simulink model "Tflex_PIDv1_ISSGP18a"  (R2018a)
settings: Solver=FixedStepDiscrete  StartTime=0.0  StopTime=inf  FixedStep=0.001  RelTol=1e-3  EnableMultiTasking=on
PreLoadFcn:
  | Ts = 0.001;
InitFcn:
  | Ts = 0.001;
values from neighbouring files (symbols this model uses):
  a0 = W_n^3    (= 31006276.6803)    [init_Tflex_PID_ISSGP.m]
  a1 = 0.5    [ADRC_lin_PAR.m]    (also in init_Tflex_PID_ISSGP.m = 296088.132033)
  a2 = 0.25    [ADRC_lin_PAR.m]    (also in init_Tflex_PID_ISSGP.m = 942.477796077)
  b = ones(2*D,Q)*0.001    [init_Tflex_PID_ISSGP.m]
  D = 20    [init_Tflex_PID_ISSGP.m]
  I_limit = 2000    [init_Tflex_PID_ISSGP.m]
  kp = m_eq*W_c^2/sqrt(1/alpha)    [init_Tflex_PID_ISSGP.m]
  mu_X = [0,0,0]    [init_Tflex_PID_ISSGP.m]
  mu_Y = 0    [init_Tflex_PID_ISSGP.m]
  R = eye(2*D,2*D)*sn    [init_Tflex_PID_ISSGP.m]
  seed = 1    [init_Tflex_PID_ISSGP.m]
  sig_Y = 1    [init_Tflex_PID_ISSGP.m]
  sp_ts = 1.5    [init_Tflex_PID_ISSGP.m]
  t_switch = 10    [init_Tflex_PID_ISSGP.m]
  tau_i = beta*tau_z    [init_Tflex_PID_ISSGP.m]
  tau_p = 1/(sqrt(1/alpha)*W_c)    [init_Tflex_PID_ISSGP.m]
  tau_z = sqrt(1/alpha)/W_c    [init_Tflex_PID_ISSGP.m]
  tm = 1    [init_Tflex_PID_ISSGP.m]
  ts = 0.001    [ADRC_lin_PAR.m]    (also in PIDtuning.m; init_Tflex_PID_ISSGP.m)
  w = ones(2*D,Q)*0.001    [init_Tflex_PID_ISSGP.m]
undefined symbols (not defined in the file or in its folder): Avout, DiscIntNeverNeededParam, FB1_offset, FF, KTY_p0, KTY_p1, sf1, sig_X, SIGMA
libraries: xpcethercatlib x17, simulink x10, slrtlib x6
settings Model: xpc_rtwmakecfg_data=_xpcethercatlib_  SimulationMode=external  ExtModeTrigDirection=either  Creator=lab  LastModifiedBy=wout7
settings SolverCC: ConcurrentTasks=on  AutoInsertRateTranBlk=on
settings DataIOCC: LimitDataPoints=on  SaveFormat=StructureWithTime
settings OptimizationCC: BlockReduction=off  OptimizeBlockIOStorage=off  BufferReuse=off  GlobalBufferReuse=off  ExpressionFolding=off  LocalBlockOutputs=off  OptimizeDataStoreBuffers=off  BusAssignmentInplaceUpdate=off
settings DebuggingCC: UnconnectedInputMsg=none  UnconnectedOutputMsg=none  UnconnectedLineMsg=none
settings HardwareCC: ProdBitPerPointer=32  ProdBitPerSizeT=32  ProdBitPerPtrDiffT=32  ProdLargestAtomicFloat=None  ProdWordSize=32  ProdLongLongMode=on  ProdHWDeviceType=Generic->32-bit x86 compatible
settings RTWCC: SystemTargetFile=slrt.tlc  TemplateMakefile=slrt_default_tmf  Description=Simulink Real-Time  CodeExecutionProfiling=on  RTWCompilerOptimization=on
settings SimulinkRealTimeCC: SupportVariableSizeSignals=on  xPCConcurrentTasks=on

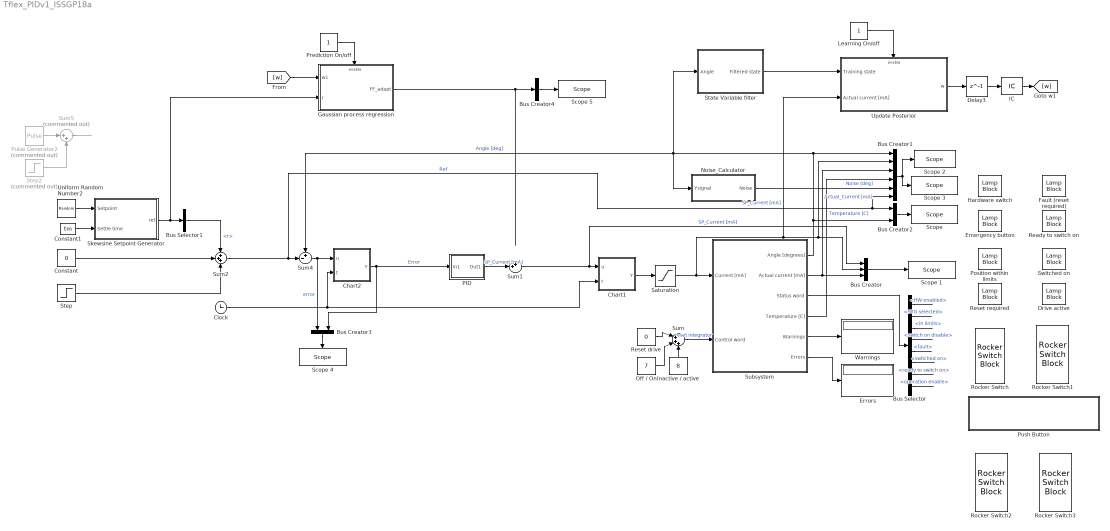
== system Tflex_PIDv1_ISSGP18a ==
  Bus Creator : BusCreator  Inputs=3
  Bus Creator1 : BusCreator  Inputs=6
  Bus Creator2 : BusCreator  Inputs=2
  Bus Creator3 : BusCreator  Inputs=2
  Bus Creator4 : BusCreator  Inputs=1
  Bus Selector : BusSelector  OutputSignals=HW enabled,STO selected,in limits,switch on disable,fault,switched on,ready to switch on,operation enable
  Bus Selector1 : BusSelector  OutputSignals=r
  Chart1 : Stateflow chart  TreatAsAtomicUnit=on
  Chart2 : Stateflow chart  TreatAsAtomicUnit=on
  Clock : Clock
  Constant : Constant  Value=0
  Constant1 : Constant  Value=tm
  Delay3 : Delay  DelayLength=1  InitialCondition=0
  Drive active : LampBlock  WebBlockId=227
  Emergency button : LampBlock  WebBlockId=221
  Errors : Display
  Fault (reset required) : LampBlock  WebBlockId=224
  Gaussian process regression : Subsystem
  Hardware switch : LampBlock  WebBlockId=218
  IC : InitialCondition  Value=w
  Inactive / active : Constant  Value=8
  Learning On/off : Constant
  Noise_Calculator : Subsystem
  Off / On : Constant  Value=7
  "PID " : Subsystem
  Position within limits : LampBlock  WebBlockId=222
  Prediction On/off : Constant
  Pulse Generator2 : DiscretePulseGenerator  Commented=on  Amplitude=80*pi/180  Period=4  PulseWidth=2  SampleTime=sp_ts
  Push Button : Subsystem  DialogController=hmiCreateDDGDialog  IsWebBlock=on  mask(MWDashboardBlock){webBlockId=9d06e9e6-678e-49a7-9d5a-3d94fac02d4b, webBlockType=pushbutton, ShowInLibBrowser=on, ShowInitialText=on, HMISrcModelName=Tflex_PIDv1_ISSGP18a}
      mask prompts: webBlockId "WebBlock Id"; webBlockType "WebBlock Type"; HMISrcModelName "Source Model"
      mask help: Set a value of a tunable parameter or variable by selecting and holding the button. When the push button is not selected, the value is set back to the default value.
      mask Help: helpview([docroot '/mapfiles/simulink.map'], 'hmi_pushbutton')
      mask Display:
      | if strcmp(get_param(bdroot(gcb),'BlockDiagramType'),'library')
      |  image([(matlabroot) '/toolbox/simulink/hmi/icons/PushButton.png'])
      | end
  Ready to switch on : LampBlock  WebBlockId=226
  Reset drive : Constant  Value=0
  Reset required : LampBlock  WebBlockId=223
  Rocker Switch : RockerSwitchBlock  WebBlockId=231
      settings: Values={{'Off', 'On'}, [6 7]}
  Rocker Switch1 : RockerSwitchBlock  WebBlockId=232
      settings: Values={{'Off', 'On'}, [0 8]}
  Rocker Switch2 : RockerSwitchBlock  WebBlockId=965
      settings: Values={{'Off', 'Learning on'}, [0 1]}
  Rocker Switch3 : RockerSwitchBlock  WebBlockId=969
      settings: Values={{'Off', 'Prediction On'}, [0 1]}
  Saturation : Saturate  UpperLimit=I_limit  LowerLimit=-I_limit
  "Scope " : slrtlib/Displays and Logging/Scope   scopeno=1  scopetype=Target  autostart=on  viewmode=Graphical redraw  formatstr='%15.6f'  grid=on  ylimits=[0 ,0]  nosamples=2000  noprepostsamples=0  interleave=1  triggermode=FreeRun  triggersignal=1  trigsignalfromport=off  triggerlevel=0.0  triggerslope=Either  triggerscope=1  triggersample=0  filename=data.dat  mode=Lazy  writesize=512  autorestart=off  dynamicfilemode=off  maxwritefilesize=512*1024^2
  Scope 1 : slrtlib/Displays and Logging/Scope   scopeno=2  scopetype=Target  autostart=on  viewmode=Graphical redraw  formatstr='%15.6f'  grid=on  ylimits=[500,500]  nosamples=250  noprepostsamples=0  interleave=1  triggermode=FreeRun  triggersignal=1  trigsignalfromport=off  triggerlevel=0.0  triggerslope=Either  triggerscope=1  triggersample=0  filename=data.dat  mode=Lazy  writesize=512  autorestart=off  dynamicfilemode=off  maxwritefilesize=512*1024^2
  Scope 2 : slrtlib/Displays and Logging/Scope   scopeno=3  scopetype=Target  autostart=on  viewmode=Numerical  formatstr='%15.6f,%15.6f,%15.6f,%15.0f'  grid=on  ylimits=[500,500]  nosamples=250  noprepostsamples=0  interleave=1  triggermode=FreeRun  triggersignal=1  trigsignalfromport=off  triggerlevel=0.0  triggerslope=Either  triggerscope=1  triggersample=0  filename=data.dat  mode=Lazy  writesize=512  autorestart=off  dynamicfilemode=off  maxwritefilesize=512*1024^2
  Scope 3 : slrtlib/Displays and Logging/Scope   scopeno=11  scopetype=File  autostart=on  viewmode=Graphical redraw  formatstr='%15.6f'  grid=on  ylimits=[0,0]  nosamples=600000  noprepostsamples=0  interleave=1  triggermode=FreeRun  triggersignal=1  trigsignalfromport=off  triggerlevel=0.0  triggerslope=Either  triggerscope=1  triggersample=0  filename=data.dat  mode=Lazy  writesize=512  autorestart=off  dynamicfilemode=off  maxwritefilesize=512*1024^2
  Scope 4 : slrtlib/Displays and Logging/Scope   scopeno=4  scopetype=Target  autostart=on  viewmode=Numerical  formatstr='%15.6f'  grid=on  ylimits=[500,500]  nosamples=250  noprepostsamples=0  interleave=1  triggermode=FreeRun  triggersignal=1  trigsignalfromport=off  triggerlevel=0.0  triggerslope=Either  triggerscope=1  triggersample=0  filename=data.dat  mode=Lazy  writesize=512  autorestart=off  dynamicfilemode=off  maxwritefilesize=512*1024^2
  Scope 5 : slrtlib/Displays and Logging/Scope   scopeno=5  scopetype=Target  autostart=on  viewmode=Graphical redraw  formatstr='%15.6f'  grid=on  ylimits=[500,500]  nosamples=250  noprepostsamples=0  interleave=1  triggermode=FreeRun  triggersignal=1  trigsignalfromport=off  triggerlevel=0.0  triggerslope=Either  triggerscope=1  triggersample=0  filename=data.dat  mode=Lazy  writesize=512  autorestart=off  dynamicfilemode=off  maxwritefilesize=512*1024^2
  Skewsine Setpoint Generator : Subsystem
  State Variable filter : Subsystem
  Step : Step  Time=20  Before=-20  After=0  SampleTime=0
  Step2 : Step  Commented=on  Time=sp_ts  After=-40*pi/180  SampleTime=sp_ts
  Subsystem : Subsystem
  Sum : Sum  Inputs=|+++
  Sum1 : Sum  Inputs=++|
  Sum2 : Sum  Inputs=+++
  Sum4 : Sum  Inputs=+-|
  Sum5 : Sum  Commented=on  Inputs=|++
  Switched on : LampBlock  WebBlockId=225
  Uniform Random Number2 : UniformRandomNumber  Minimum=-10*pi/180  Maximum=10*pi/180  Seed=seed  SampleTime=sp_ts
  Update Posterior : Subsystem
  Warnings : Display
  wires:
  Subsystem/2(Actual current [mA]) -> Bus Creator1/3, Bus Creator/3  "Actual_Current [mA]"
  Subsystem/3(Status word) -> Bus Selector/1
  Bus Selector/1 -> ?  "<HW enabled>"
  Bus Selector/2 -> ?  "<STO selected>"
  Bus Selector/3 -> ?  "<in limits>"
  Bus Selector/4 -> ?  "<switch on disable>"
  Bus Selector/5 -> ?  "<fault>"
  Bus Selector/6 -> ?  "<switched on>"
  Bus Selector/7 -> ?  "<ready to switch on>"
  Bus Selector/8 -> ?  "<operation enable>"
  Reset drive/1 -> Sum/1
  Off / On/1 -> Sum/2
  Inactive / active/1 -> Sum/3
  Bus Creator/1 -> Scope 1/1
  Bus Creator1/1 -> Scope 2/1, Scope 3/1
  Subsystem/4(Temperature [C]) -> Bus Creator1/4  "Temperature [C]"
  Subsystem/5(Warnings) -> Warnings/1
  Subsystem/6(Errors) -> Errors/1
  Saturation/1 -> Bus Creator1/2, Bus Creator/2, Update Posterior/2("Actual current [mA] "), Subsystem/1(Current [mA])  "SP_Current [mA]"
  Sum/1 -> Subsystem/2(Control word)  "reset integrator"
  Bus Creator2/1 -> "Scope "/1
  Subsystem/1(Angle [degrees]) -> State Variable filter/1(Angle), Noise_Calculator/1(Ysignal), Sum4/1, Bus Creator1/1, Bus Creator2/2  "Angle [deg]"
  Chart1/1(Y) -> Saturation/1
  Constant/1 -> Sum2/2
  Sum1/1 -> Bus Creator/1, Chart1/1(u)  "SP_Current [mA]"
  Chart2/1(Y) -> "PID "/1(In1), Bus Creator3/2  "Error"
  Sum4/1 -> Chart2/1(u), Bus Creator3/1  "error"
  Clock/1 -> Chart1/2(t), Chart2/2(t)
  Sum2/1 -> Bus Creator1/6, Bus Creator2/1, Sum4/2  "Ref"
  Bus Creator3/1 -> Scope 4/1
  Noise_Calculator/1(Noise) -> Bus Creator1/5  "Noise [deg]"
  State Variable filter/1(Filtered state) -> Update Posterior/1(Training state)
  IC/1 -> [w]
  Delay3/1 -> IC/1
  Update Posterior/1(w) -> Delay3/1
  [w] -> Gaussian process regression/1(w1)
  Uniform Random Number2/1 -> Skewsine Setpoint Generator/1(Setpoint)
  Step/1 -> Sum2/3
  Skewsine Setpoint Generator/1(ref) -> Gaussian process regression/2(r), Bus Selector1/1
  Bus Selector1/1 -> Sum2/1  "<r>"
  "PID "/1(Out1) -> Sum1/2  "SP_Current [mA]"
  Prediction On/off/1 -> Gaussian process regression/Enable
  Learning On/off/1 -> Update Posterior/Enable
  Bus Creator4/1 -> Scope 5/1
  Gaussian process regression/1(FF_adapt) -> Bus Creator4/1
  Constant1/1 -> Skewsine Setpoint Generator/2(Settle time)
  Sum5/1 -> ?
  Step2/1 -> Sum5/2
  Pulse Generator2/1 -> Sum5/1

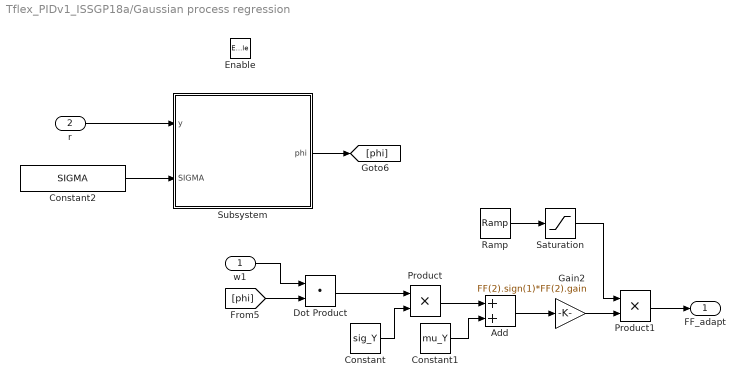
== system Tflex_PIDv1_ISSGP18a/Gaussian process regression ==
  w1 : Inport
  r : Inport  Port=2
  Enable : EnablePort
  Add : Sum
  Constant : Constant  Value=sig_Y  VectorParams1D=off
  Constant1 : Constant  Value=mu_Y  VectorParams1D=off
  Constant2 : Constant  Value=SIGMA  VectorParams1D=off  SampleTime=-1
  Dot Product : DotProduct  OutDataTypeStr=Inherit: Inherit via internal rule
  Gain2 : Gain  Gain=FF(2).sign(1)*FF(2).gain
  Product : Product
  Product1 : Product
  Ramp : simulink/Sources/Ramp  slope=1/t_switch  start=t_predict  InitialOutput=0
  Saturation : Saturate  UpperLimit=1  LowerLimit=0
  Subsystem : Subsystem
  FF_adapt : Outport
  wires:
  w1/1 -> Dot Product/1
  [phi] -> Dot Product/2
  Constant2/1 -> Subsystem/2(SIGMA)
  Subsystem/1(phi) -> [phi]
  Constant/1 -> Product/2
  Dot Product/1 -> Product/1
  Add/1 -> Gain2/1
  Product/1 -> Add/1
  Constant1/1 -> Add/2
  r/1 -> Subsystem/1(y)
  Ramp/1 -> Saturation/1
  Gain2/1 -> Product1/2
  Saturation/1 -> Product1/1
  Product1/1 -> FF_adapt/1

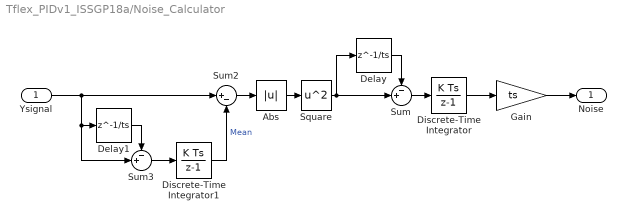
== system Tflex_PIDv1_ISSGP18a/Noise_Calculator ==
  Ysignal : Inport
  Abs : Abs
  Delay : Delay  DelayLength=1/ts  SampleTime=ts
  Delay1 : Delay  DelayLength=1/ts
  Discrete-Time Integrator : DiscreteIntegrator  gainval=1  SampleTime=ts  ICPrevOutput=DiscIntNeverNeededParam  ICPrevScaledInput=DiscIntNeverNeededParam
  Discrete-Time Integrator1 : DiscreteIntegrator  gainval=1  SampleTime=ts  ICPrevOutput=DiscIntNeverNeededParam  ICPrevScaledInput=DiscIntNeverNeededParam
  Gain : Gain  Gain=ts
  Square : Math  Operator=square  SaturateOnIntegerOverflow=on
  Sum : Sum  Inputs=-+|
  Sum2 : Sum  Inputs=|+-
  Sum3 : Sum  Inputs=-+|
  Noise : Outport
  wires:
  Ysignal/1 -> Sum2/1, Sum3/2, Delay1/1
  Delay1/1 -> Sum3/1
  Sum2/1 -> Abs/1
  Abs/1 -> Square/1
  Discrete-Time Integrator1/1 -> Sum2/2  "Mean"
  Sum/1 -> Discrete-Time Integrator/1
  Discrete-Time Integrator/1 -> Gain/1
  Square/1 -> Delay/1, Sum/2
  Delay/1 -> Sum/1
  Sum3/1 -> Discrete-Time Integrator1/1
  Gain/1 -> Noise/1

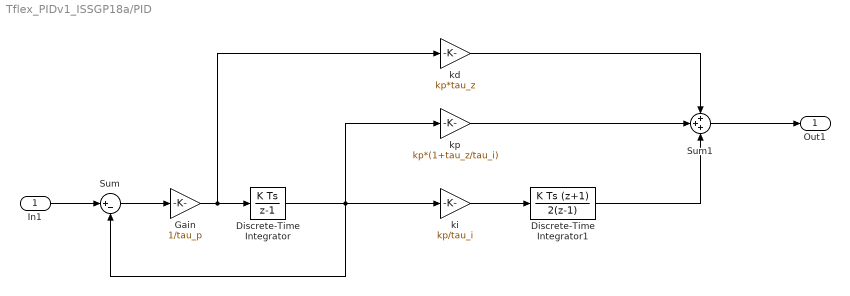
== system Tflex_PIDv1_ISSGP18a/PID  ==
  In1 : Inport
  Discrete-Time Integrator : DiscreteIntegrator  SampleTime=ts  ICPrevOutput=DiscIntNeverNeededParam  ICPrevScaledInput=DiscIntNeverNeededParam
  Discrete-Time Integrator1 : DiscreteIntegrator  IntegratorMethod=Integration: Trapezoidal  SampleTime=ts  LimitOutput=on  UpperSaturationLimit=I_limit  LowerSaturationLimit=-I_limit  ICPrevOutput=DiscIntNeverNeededParam  ICPrevScaledInput=DiscIntNeverNeededParam
  Gain : Gain  Gain=1/tau_p
  Sum : Sum  Inputs=|+-
  Sum1 : Sum  Inputs=+++
  kd : Gain  Gain=kp*tau_z
  ki : Gain  Gain=kp/tau_i
  kp : Gain  Gain=kp*(1+tau_z/tau_i)
  Out1 : Outport
  wires:
  In1/1 -> Sum/1
  Sum/1 -> Gain/1
  Gain/1 -> kd/1, Discrete-Time Integrator/1
  Discrete-Time Integrator/1 -> kp/1, ki/1, Sum/2
  kp/1 -> Sum1/2
  kd/1 -> Sum1/1
  ki/1 -> Discrete-Time Integrator1/1
  Sum1/1 -> Out1/1
  Discrete-Time Integrator1/1 -> Sum1/3

== system Tflex_PIDv1_ISSGP18a/Push Button ==

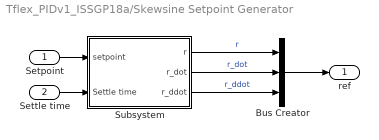
== system Tflex_PIDv1_ISSGP18a/Skewsine Setpoint Generator ==
  Setpoint : Inport
  Settle time : Inport  Port=2
  Bus Creator : BusCreator  Inputs=3
  Subsystem : Subsystem
  ref : Outport
  wires:
  Subsystem/3(r_ddot) -> Bus Creator/3  "r_ddot"
  Bus Creator/1 -> ref/1
  Setpoint/1 -> Subsystem/1(setpoint)
  Subsystem/2(r_dot) -> Bus Creator/2  "r_dot"
  Subsystem/1(r) -> Bus Creator/1  "r"
  Settle time/1 -> Subsystem/2(Settle time)

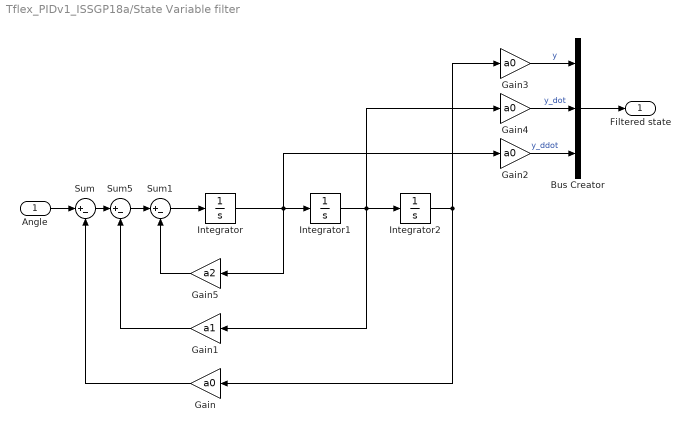
== system Tflex_PIDv1_ISSGP18a/State Variable filter ==
  Angle : Inport
  Bus Creator : BusCreator  Inputs=3
  Gain{,2..4} (4 alike) : Gain  Gain=a0
  Gain1 : Gain  Gain=a1
  Gain5 : Gain  Gain=a2
  Integrator : Integrator  UpperSaturationLimit=1  LowerSaturationLimit=-1
  Integrator1 : Integrator
  Integrator2 : Integrator
  Sum : Sum  Inputs=|+-
  Sum1 : Sum  Inputs=|+-
  Sum5 : Sum  Inputs=|+-
  Filtered state : Outport
  wires:
  Bus Creator/1 -> Filtered state/1
  Sum1/1 -> Integrator/1
  Angle/1 -> Sum/1
  Sum/1 -> Sum5/1
  Gain/1 -> Sum/2
  Gain1/1 -> Sum5/2
  Gain3/1 -> Bus Creator/1  "y"
  Gain2/1 -> Bus Creator/3  "y_ddot"
  Gain4/1 -> Bus Creator/2  "y_dot"
  Gain5/1 -> Sum1/2
  Sum5/1 -> Sum1/1
  Integrator/1 -> Gain2/1, Integrator1/1, Gain5/1
  Integrator1/1 -> Gain4/1, Integrator2/1, Gain1/1
  Integrator2/1 -> Gain3/1, Gain/1

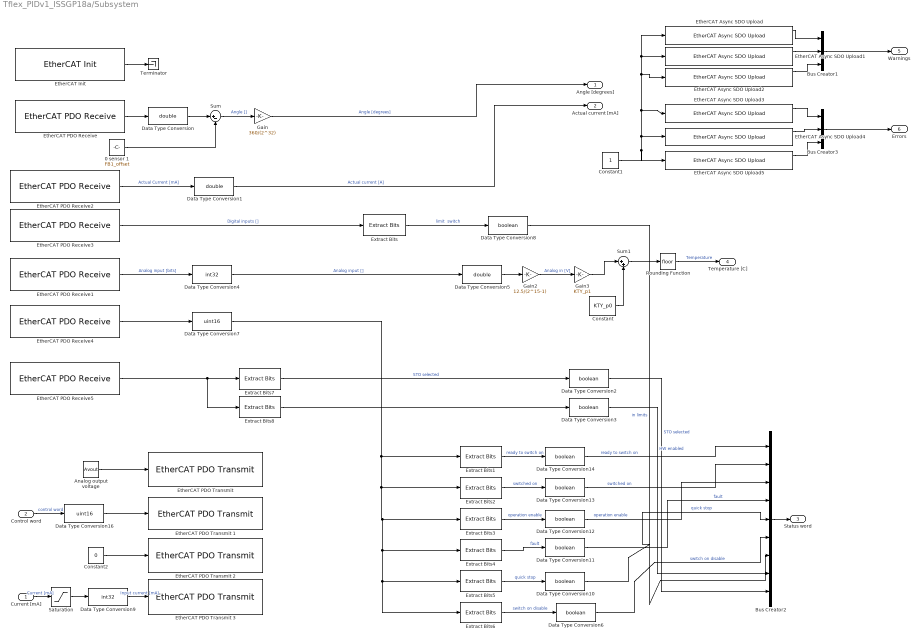
== system Tflex_PIDv1_ISSGP18a/Subsystem ==
  Current [mA] : Inport
  Control word : Inport  Port=2
  0 sensor 1 : Constant  Value=FB1_offset
  Analog output voltage : Constant  Value=Avout  OutDataTypeStr=int16
  Bus Creator1 : BusCreator  Inputs=3
  Bus Creator2 : BusCreator  Inputs=9
  Bus Creator3 : BusCreator  Inputs=3
  Constant : Constant  Value=KTY_p0
  Constant1 : Constant  OutDataTypeStr=int32
  Constant2 : Constant  Value=0  OutDataTypeStr=uint32
  Data Type Conversion : DataTypeConversion  OutDataTypeStr=double
  Data Type Conversion1 : DataTypeConversion  OutDataTypeStr=double
  Data Type Conversion{2..3,6,8,10..14} (9 alike) : DataTypeConversion  OutDataTypeStr=boolean
  Data Type Conversion16 : DataTypeConversion  OutDataTypeStr=uint16
  Data Type Conversion4 : DataTypeConversion  OutDataTypeStr=int32
  Data Type Conversion5 : DataTypeConversion  OutDataTypeStr=double
  Data Type Conversion7 : DataTypeConversion  OutDataTypeStr=uint16  RndMeth=Round
  Data Type Conversion9 : DataTypeConversion  OutDataTypeStr=int32
  EtherCAT Async SDO Upload : xpcethercatlib/EtherCAT Async SDO Upload  index=8192  subIndex=1  sig_type=uint32  sig_dim=1  device_id=0  slave_name=Drive 1 (AKD)  sample_time=1  slave_addr=1001  selected_slave=Term 1 (EK1100)  timeout=500  slave_found=1
      settings: SourceProductName=Simulink Real-Time  SourceProductBaseCode=XP
  EtherCAT Async SDO Upload1 : xpcethercatlib/EtherCAT Async SDO Upload  index=8192  subIndex=2  sig_type=uint32  sig_dim=1  device_id=0  slave_name=Drive 1 (AKD)  sample_time=1  slave_addr=1001  selected_slave=Term 1 (EK1100)  timeout=500  slave_found=1
      settings: SourceProductName=Simulink Real-Time  SourceProductBaseCode=XP
  EtherCAT Async SDO Upload2 : xpcethercatlib/EtherCAT Async SDO Upload  index=8192  subIndex=3  sig_type=uint32  sig_dim=1  device_id=0  slave_name=Drive 1 (AKD)  sample_time=1  slave_addr=1001  selected_slave=Term 1 (EK1100)  timeout=500  slave_found=1
      settings: SourceProductName=Simulink Real-Time  SourceProductBaseCode=XP
  EtherCAT Async SDO Upload3 : xpcethercatlib/EtherCAT Async SDO Upload  index=8193  subIndex=1  sig_type=uint32  sig_dim=1  device_id=0  slave_name=Drive 1 (AKD)  sample_time=1  slave_addr=1001  selected_slave=Term 1 (EK1100)  timeout=500  slave_found=1
      settings: SourceProductName=Simulink Real-Time  SourceProductBaseCode=XP
  EtherCAT Async SDO Upload4 : xpcethercatlib/EtherCAT Async SDO Upload  index=8193  subIndex=2  sig_type=uint32  sig_dim=1  device_id=0  slave_name=Drive 1 (AKD)  sample_time=1  slave_addr=1001  selected_slave=Term 1 (EK1100)  timeout=500  slave_found=1
      settings: SourceProductName=Simulink Real-Time  SourceProductBaseCode=XP
  EtherCAT Async SDO Upload5 : xpcethercatlib/EtherCAT Async SDO Upload  index=8193  subIndex=3  sig_type=uint32  sig_dim=1  device_id=0  slave_name=Drive 1 (AKD)  sample_time=1  slave_addr=1001  selected_slave=Term 1 (EK1100)  timeout=500  slave_found=1
      settings: SourceProductName=Simulink Real-Time  SourceProductBaseCode=XP
  "EtherCAT Init " : xpcethercatlib/EtherCAT Init   Priority=0  config_file=C:\Users\Mark\Desktop\tflex\simulink\custom_pdo_eni3.xml  device_id=0  pci_bus=13  pci_slot=0  pci_function=0  initstate=2  dctuning=0  enaDebug=off  enaDC=on  errLink=off  masterDbg=off  stateChgDbg=off  baseClock=off  masterCfg=off  logFile='c:\dbglog.txt'  sample_time=0.001000  DCMode=2
      settings: SourceProductName=Simulink Real-Time  SourceProductBaseCode=XP
  EtherCAT PDO Receive : xpcethercatlib/EtherCAT PDO Receive  Priority=2  sig_name=Drive 1 (AKD).TPDO mapping parameter 3.Position actual internal value  sig_offset=624  sig_type=int32  type_size=32  sig_dim=1  device_id=0  sample_time=0.001000
      settings: SourceProductName=Simulink Real-Time  SourceProductBaseCode=XP
  EtherCAT PDO Receive1 : xpcethercatlib/EtherCAT PDO Receive  Priority=2  sig_name=Drive 1 (AKD).TPDO mapping parameter 1.AOUT_INPUT_VALUE  sig_offset=480  sig_type=int16  type_size=16  sig_dim=1  device_id=0  sample_time=0.001000
      settings: SourceProductName=Simulink Real-Time  SourceProductBaseCode=XP
  EtherCAT PDO Receive2 : xpcethercatlib/EtherCAT PDO Receive  Priority=2  sig_name=Drive 1 (AKD).TPDO mapping parameter 2.Current actual value  sig_offset=528  sig_type=int32  type_size=32  sig_dim=1  device_id=0  sample_time=0.001000
      settings: SourceProductName=Simulink Real-Time  SourceProductBaseCode=XP
  EtherCAT PDO Receive3 : xpcethercatlib/EtherCAT PDO Receive  Priority=2  sig_name=Drive 1 (AKD).TPDO mapping parameter 1.Digital inputs  sig_offset=496  sig_type=uint32  type_size=32  sig_dim=1  device_id=0  sample_time=0.001000
      settings: SourceProductName=Simulink Real-Time  SourceProductBaseCode=XP
  EtherCAT PDO Receive4 : xpcethercatlib/EtherCAT PDO Receive  Priority=2  sig_name=Drive 1 (AKD).TPDO mapping parameter 1.Statusword  sig_offset=464  sig_type=uint16  type_size=16  sig_dim=1  device_id=0  sample_time=0.001000
      settings: SourceProductName=Simulink Real-Time  SourceProductBaseCode=XP
  EtherCAT PDO Receive5 : xpcethercatlib/EtherCAT PDO Receive  Priority=2  sig_name=Drive 1 (AKD).TPDO mapping parameter 3.Manufacturer status register  sig_offset=592  sig_type=uint32  type_size=32  sig_dim=1  device_id=0  sample_time=0.001000
      settings: SourceProductName=Simulink Real-Time  SourceProductBaseCode=XP
  "EtherCAT PDO Transmit " : xpcethercatlib/EtherCAT PDO Transmit   Priority=3  sig_name=Drive 1 (AKD).RPDO mapping parameter 1.AOUT.VALUE write  sig_offset=480  sig_type=int16  type_size=16  sig_dim=1  device_id=0  sample_time=0.001000
      settings: SourceProductName=Simulink Real-Time  SourceProductBaseCode=XP
  EtherCAT PDO Transmit 1 : xpcethercatlib/EtherCAT PDO Transmit   Priority=3  sig_name=Drive 1 (AKD).RPDO mapping parameter 1.Controlword  sig_offset=464  sig_type=uint16  type_size=16  sig_dim=1  device_id=0  sample_time=0.001000
      settings: SourceProductName=Simulink Real-Time  SourceProductBaseCode=XP
  EtherCAT PDO Transmit 2 : xpcethercatlib/EtherCAT PDO Transmit   Priority=3  sig_name=Drive 1 (AKD).RPDO mapping parameter 1.Physical outputs  sig_offset=496  sig_type=uint32  type_size=32  sig_dim=1  device_id=0  sample_time=0.001000
      settings: SourceProductName=Simulink Real-Time  SourceProductBaseCode=XP
  EtherCAT PDO Transmit 3 : xpcethercatlib/EtherCAT PDO Transmit   Priority=3  sig_name=Drive 1 (AKD).RPDO mapping parameter 2.Target current  sig_offset=528  sig_type=int32  type_size=32  sig_dim=1  device_id=0  sample_time=0.001000
      settings: SourceProductName=Simulink Real-Time  SourceProductBaseCode=XP
  Extract Bits : simulink/Logic and Bit Operations/Extract Bits  bitsToExtract=Range of bits  numBits=8  bitIdxRange=[16]  outScalingMode=Treat bit field as an integer
      settings: SourceProductName=Simulink
  Extract Bits1 : simulink/Logic and Bit Operations/Extract Bits  bitsToExtract=Range of bits  numBits=8  bitIdxRange=[0]  outScalingMode=Treat bit field as an integer
      settings: SourceProductName=Simulink
  Extract Bits2 : simulink/Logic and Bit Operations/Extract Bits  bitsToExtract=Range of bits  numBits=8  bitIdxRange=[1]  outScalingMode=Treat bit field as an integer
      settings: SourceProductName=Simulink
  Extract Bits3 : simulink/Logic and Bit Operations/Extract Bits  bitsToExtract=Range of bits  numBits=8  bitIdxRange=[2]  outScalingMode=Treat bit field as an integer
      settings: SourceProductName=Simulink
  Extract Bits4 : simulink/Logic and Bit Operations/Extract Bits  bitsToExtract=Range of bits  numBits=8  bitIdxRange=[3]  outScalingMode=Treat bit field as an integer
      settings: SourceProductName=Simulink
  Extract Bits5 : simulink/Logic and Bit Operations/Extract Bits  bitsToExtract=Range of bits  numBits=8  bitIdxRange=[5]  outScalingMode=Treat bit field as an integer
      settings: SourceProductName=Simulink
  Extract Bits6 : simulink/Logic and Bit Operations/Extract Bits  bitsToExtract=Range of bits  numBits=8  bitIdxRange=[6]  outScalingMode=Treat bit field as an integer
      settings: SourceProductName=Simulink
  Extract Bits7 : simulink/Logic and Bit Operations/Extract Bits  bitsToExtract=Range of bits  numBits=8  bitIdxRange=[13]  outScalingMode=Treat bit field as an integer
      settings: SourceProductName=Simulink
  Extract Bits8 : simulink/Logic and Bit Operations/Extract Bits  bitsToExtract=Range of bits  numBits=8  bitIdxRange=[29]  outScalingMode=Treat bit field as an integer
      settings: SourceProductName=Simulink
  Gain : Gain  Gain=360/(2^32)
  Gain2 : Gain  Gain=12.5/(2^15-1)
  Gain3 : Gain  Gain=KTY_p1
  Rounding Function : Rounding
  Saturation : Saturate  UpperLimit=I_limit  LowerLimit=-I_limit
  Sum : Sum  Inputs=|+-
  Sum1 : Sum  Inputs=|++  OutDataTypeStr=double
  Terminator : Terminator
  Angle [degrees] : Outport
  Actual current [mA] : Outport  Port=2
  Status word : Outport  Port=3
  Temperature [C] : Outport  Port=4
  Warnings : Outport  Port=5
  Errors : Outport  Port=6
  wires:
  Data Type Conversion/1 -> Sum/1
  Data Type Conversion9/1 -> EtherCAT PDO Transmit 3/1  "Input current [mA]"
  Bus Creator2/1 -> Status word/1
  0 sensor 1/1 -> Sum/2
  Data Type Conversion1/1 -> Actual current [mA]/1  "Actual current [A]"
  Data Type Conversion7/1 -> Extract Bits1/1, Extract Bits2/1, Extract Bits3/1, Extract Bits4/1, Extract Bits5/1, Extract Bits6/1
  EtherCAT PDO Receive4/1 -> Data Type Conversion7/1
  EtherCAT PDO Receive2/1 -> Data Type Conversion1/1  "Actual Current [mA]"
  Data Type Conversion4/1 -> Data Type Conversion5/1  "Analog input []"
  EtherCAT PDO Receive/1 -> Data Type Conversion/1
  Gain/1 -> Angle [degrees]/1  "Angle [degrees]"
  EtherCAT PDO Receive5/1 -> Extract Bits8/1, Extract Bits7/1
  EtherCAT PDO Receive1/1 -> Data Type Conversion4/1  "Analog input [bits]"
  Sum/1 -> Gain/1  "Angle []"
  Data Type Conversion8/1 -> Bus Creator2/7  "in limits"
  Data Type Conversion3/1 -> Bus Creator2/8  "HW enabled"
  Control word/1 -> Data Type Conversion16/1  "control word"
  Extract Bits8/1 -> Data Type Conversion3/1
  Extract Bits6/1 -> Data Type Conversion6/1  "switch on disable"
  Data Type Conversion13/1 -> Bus Creator2/2  "switched on"
  Data Type Conversion6/1 -> Bus Creator2/6  "switch on disable"
  Data Type Conversion12/1 -> Bus Creator2/3  "operation enable"
  Extract Bits/1 -> Data Type Conversion8/1  "limit  switch"
  Extract Bits3/1 -> Data Type Conversion12/1  "operation enable"
  Extract Bits2/1 -> Data Type Conversion13/1  "switched on"
  Data Type Conversion11/1 -> Bus Creator2/4  "fault"
  Extract Bits4/1 -> Data Type Conversion11/1  "fault"
  Data Type Conversion10/1 -> Bus Creator2/5  "quick stop"
  Extract Bits5/1 -> Data Type Conversion10/1  "quick stop"
  Data Type Conversion14/1 -> Bus Creator2/1  "ready to switch on"
  Constant2/1 -> EtherCAT PDO Transmit 2/1
  Extract Bits1/1 -> Data Type Conversion14/1  "ready to switch on"
  EtherCAT PDO Receive3/1 -> Extract Bits/1  "Digital inputs []"
  Data Type Conversion2/1 -> Bus Creator2/9  "STO selected"
  Extract Bits7/1 -> Data Type Conversion2/1  "STO selected"
  Current [mA]/1 -> Saturation/1  "Current [mA]"
  Data Type Conversion16/1 -> EtherCAT PDO Transmit 1/1
  "EtherCAT Init "/1 -> Terminator/1
  Data Type Conversion5/1 -> Gain2/1
  Analog output voltage/1 -> "EtherCAT PDO Transmit "/1
  Gain2/1 -> Gain3/1  "Analog in [V]"
  Sum1/1 -> Rounding Function/1
  Rounding Function/1 -> Temperature [C]/1  "Temperature"
  EtherCAT Async SDO Upload/1 -> Bus Creator1/1
  Bus Creator1/1 -> Warnings/1
  Constant1/1 -> EtherCAT Async SDO Upload5/1, EtherCAT Async SDO Upload3/1, EtherCAT Async SDO Upload2/1, EtherCAT Async SDO Upload1/1, EtherCAT Async SDO Upload/1, EtherCAT Async SDO Upload4/1
  EtherCAT Async SDO Upload1/1 -> Bus Creator1/2
  EtherCAT Async SDO Upload2/1 -> Bus Creator1/3
  EtherCAT Async SDO Upload3/1 -> Bus Creator3/1
  EtherCAT Async SDO Upload4/1 -> Bus Creator3/2
  EtherCAT Async SDO Upload5/1 -> Bus Creator3/3
  Bus Creator3/1 -> Errors/1
  Saturation/1 -> Data Type Conversion9/1
  Gain3/1 -> Sum1/1
  Constant/1 -> Sum1/2

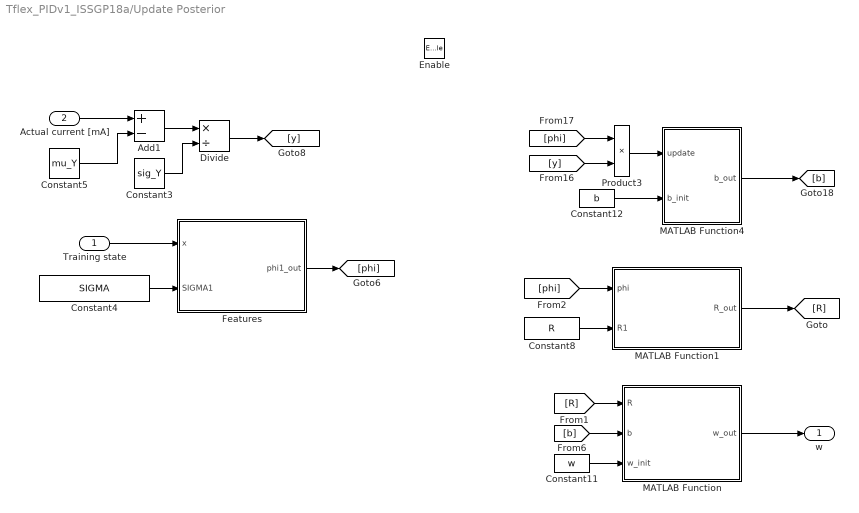
== system Tflex_PIDv1_ISSGP18a/Update Posterior ==
  Training state : Inport
  "Actual current [mA] " : Inport  Port=2
  Enable : EnablePort
  Add1 : Sum  Inputs=+-
  Constant11 : Constant  Value=w  VectorParams1D=off  SampleTime=ts
  Constant12 : Constant  Value=b  VectorParams1D=off  SampleTime=ts
  Constant3 : Constant  Value=sig_Y  VectorParams1D=off
  Constant4 : Constant  Value=SIGMA  VectorParams1D=off
  Constant5 : Constant  Value=mu_Y  VectorParams1D=off
  Constant8 : Constant  Value=R  VectorParams1D=off  SampleTime=ts
  Divide : Product  Inputs=*/
  Features : Subsystem
  MATLAB Function : MATLAB Function  TreatAsAtomicUnit=on
  MATLAB Function1 : MATLAB Function  TreatAsAtomicUnit=on
  MATLAB Function4 : MATLAB Function  TreatAsAtomicUnit=on
  Product3 : Product
  w : Outport
  wires:
  [phi] -> MATLAB Function1/1(phi)
  Training state/1 -> Features/1(x)
  Features/1(phi1_out) -> [phi]
  MATLAB Function1/1(R_out) -> [R]
  Constant4/1 -> Features/2(SIGMA1)
  "Actual current [mA] "/1 -> Add1/1
  Constant3/1 -> Divide/2
  Constant5/1 -> Add1/2
  Divide/1 -> [y]
  Add1/1 -> Divide/1
  [R] -> MATLAB Function/1(R)
  [b] -> MATLAB Function/2(b)
  MATLAB Function/1(w_out) -> w/1
  Constant8/1 -> MATLAB Function1/2(R1)
  Constant11/1 -> MATLAB Function/3(w_init)
  [y] -> Product3/2
  [phi] -> Product3/1
  Product3/1 -> MATLAB Function4/1(update)
  Constant12/1 -> MATLAB Function4/2(b_init)
  MATLAB Function4/1(b_out) -> [b]

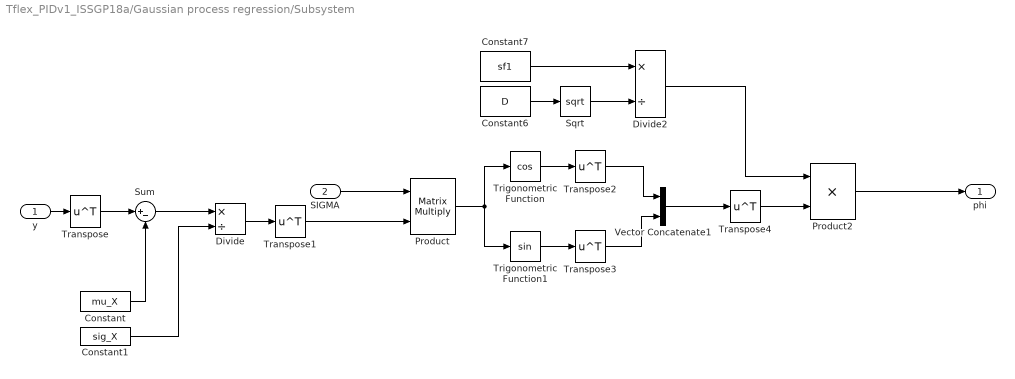
== system Tflex_PIDv1_ISSGP18a/Gaussian process regression/Subsystem ==
  y : Inport
  SIGMA : Inport  Port=2
  Constant : Constant  Value=mu_X  VectorParams1D=off  SampleTime=-1
  Constant1 : Constant  Value=sig_X  VectorParams1D=off  SampleTime=-1
  Constant6 : Constant  Value=D  SampleTime=-1
  Constant7 : Constant  Value=sf1  SampleTime=-1
  Divide : Product  Inputs=*/
  Divide2 : Product  Inputs=*/
  Product : Product  Multiplication=Matrix(*)
  Product2 : Product
  Sqrt : Sqrt  SaturateOnIntegerOverflow=on
  Sum : Sum  Inputs=|+-
  Transpose{,1..4} (5 alike) : Math  Operator=transpose  SaturateOnIntegerOverflow=on
  Trigonometric Function : Trigonometry  Operator=cos
  Trigonometric Function1 : Trigonometry
  Vector Concatenate1 : Concatenate
  phi : Outport
  wires:
  Transpose1/1 -> Product/2
  Divide/1 -> Transpose1/1
  y/1 -> Transpose/1
  Product/1 -> Trigonometric Function1/1, Trigonometric Function/1
  Product2/1 -> phi/1
  Constant7/1 -> Divide2/1
  Divide2/1 -> Product2/1
  Sum/1 -> Divide/1
  Constant1/1 -> Divide/2
  Constant/1 -> Sum/2
  Transpose2/1 -> Vector Concatenate1/1
  Transpose4/1 -> Product2/2
  Constant6/1 -> Sqrt/1
  Trigonometric Function1/1 -> Transpose3/1
  Trigonometric Function/1 -> Transpose2/1
  Vector Concatenate1/1 -> Transpose4/1
  Transpose3/1 -> Vector Concatenate1/2
  Sqrt/1 -> Divide2/2
  SIGMA/1 -> Product/1
  Transpose/1 -> Sum/1

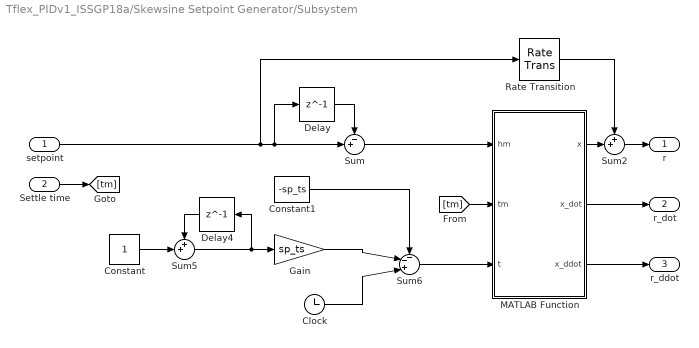
== system Tflex_PIDv1_ISSGP18a/Skewsine Setpoint Generator/Subsystem ==
  setpoint : Inport
  Settle time : Inport  Port=2
  Clock : Clock
  Constant : Constant
  Constant1 : Constant  Value=-sp_ts
  Delay : Delay  DelayLength=1  InitialCondition=0  SampleTime=sp_ts
  Delay4 : Delay  DelayLength=1  InitialCondition=0  SampleTime=sp_ts
  Gain : Gain  Gain=sp_ts
  MATLAB Function : MATLAB Function  TreatAsAtomicUnit=on
  Rate Transition : RateTransition
  Sum : Sum  Inputs=-+|
  Sum2 : Sum  Inputs=++|
  Sum5 : Sum  Inputs=++|
  Sum6 : Sum  Inputs=--+|
  r : Outport
  r_dot : Outport  Port=2
  r_ddot : Outport  Port=3
  wires:
  [tm] -> MATLAB Function/2(tm)
  MATLAB Function/1(x) -> Sum2/2
  Rate Transition/1 -> Sum2/1
  Delay4/1 -> Sum5/1
  Sum/1 -> MATLAB Function/1(hm)
  setpoint/1 -> Rate Transition/1, Delay/1, Sum/2
  Sum2/1 -> r/1
  Sum5/1 -> Delay4/1, Gain/1
  Constant/1 -> Sum5/2
  MATLAB Function/3(x_ddot) -> r_ddot/1
  Clock/1 -> Sum6/3
  Sum6/1 -> MATLAB Function/3(t)
  Delay/1 -> Sum/1
  Gain/1 -> Sum6/2
  Constant1/1 -> Sum6/1
  MATLAB Function/2(x_dot) -> r_dot/1
  Settle time/1 -> [tm]

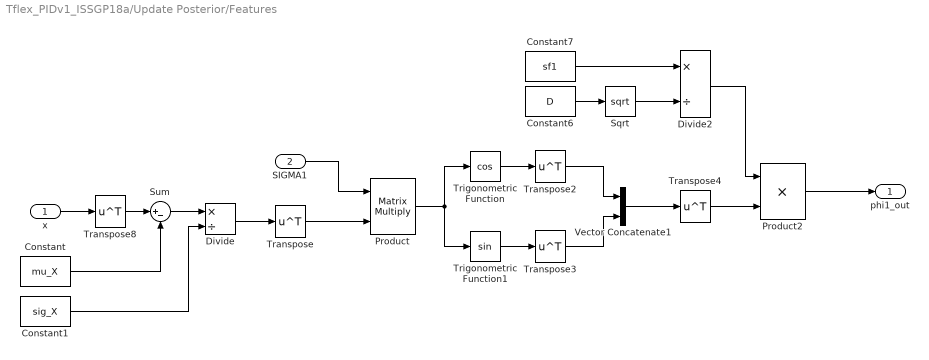
== system Tflex_PIDv1_ISSGP18a/Update Posterior/Features ==
  x : Inport
  SIGMA1 : Inport  Port=2
  Constant : Constant  Value=mu_X  VectorParams1D=off
  Constant1 : Constant  Value=sig_X  VectorParams1D=off
  Constant6 : Constant  Value=D  SampleTime=-1
  Constant7 : Constant  Value=sf1  SampleTime=-1
  Divide : Product  Inputs=*/
  Divide2 : Product  Inputs=*/
  Product : Product  Multiplication=Matrix(*)
  Product2 : Product
  Sqrt : Sqrt  SaturateOnIntegerOverflow=on
  Sum : Sum  Inputs=|+-
  Transpose{,2..4,8} (5 alike) : Math  Operator=transpose  SaturateOnIntegerOverflow=on
  Trigonometric Function : Trigonometry  Operator=cos
  Trigonometric Function1 : Trigonometry
  Vector Concatenate1 : Concatenate
  phi1_out : Outport
  wires:
  Sum/1 -> Divide/1
  SIGMA1/1 -> Product/1
  Product2/1 -> phi1_out/1
  Constant6/1 -> Sqrt/1
  Trigonometric Function1/1 -> Transpose3/1
  Trigonometric Function/1 -> Transpose2/1
  Constant7/1 -> Divide2/1
  Vector Concatenate1/1 -> Transpose4/1
  Transpose3/1 -> Vector Concatenate1/2
  Product/1 -> Trigonometric Function1/1, Trigonometric Function/1
  Constant1/1 -> Divide/2
  Transpose/1 -> Product/2
  Divide/1 -> Transpose/1
  Divide2/1 -> Product2/1
  Transpose4/1 -> Product2/2
  Sqrt/1 -> Divide2/2
  Constant/1 -> Sum/2
  Transpose2/1 -> Vector Concatenate1/1
  x/1 -> Transpose8/1
  Transpose8/1 -> Sum/1

== stateflow chart Tflex_PIDv1_ISSGP18a/Chart2 ==
  state ON
    Y=0;
  state OFF
    Y=0;
  state OFF1
    Y=u;
  (default) -> ON
  ON -> OFF : [u<90]
  OFF -> OFF1 [order 2] : [t>10]
  OFF -> ON [order 1] : [u>90]
  OFF1 -> OFF : [u>90]
  data: u input; Y output; t input

== matlab function Tflex_PIDv1_ISSGP18a/Update Posterior/MATLAB Function ==
  settings: updateMethod=DISCRETE  sampleTime=ts
  data: R input; w_out output; b input; w_init input
function w_out = updateW(R,b,w_init) %#codegen
persistent w
if(isempty(w))
    w = w_init;
end
coder.extrinsic('solve_chol');
w = solve_chol(R,b);
%w = R\(R'\b);
w_out = w;

== stateflow chart Tflex_PIDv1_ISSGP18a/Chart1 ==
  state OFF2
    Y=0;
  state ON
    Y=u;
  (default) -> OFF2
  OFF2 -> ON : [t>10]
  ON -> OFF2 : [t<10]
  data: u input; Y output; t input

== matlab function Tflex_PIDv1_ISSGP18a/Update Posterior/MATLAB Function1 ==
  settings: updateMethod=DISCRETE  sampleTime=ts
  data: R_out output; phi input; R1 input
function R_out = cholupdate_fcn(phi,R1)
persistent R; 
if(isempty(R))
    R = R1;
end
R = cholupdate(R,phi);
R_out = R;

== matlab function Tflex_PIDv1_ISSGP18a/Update Posterior/MATLAB Function4 ==
  settings: updateMethod=DISCRETE  sampleTime=ts
  data: update input; b_out output; b_init input
function b_out = fcn(update, b_init)
persistent b 
if(isempty(b))
    b = b_init;
end

b = b + update;
b_out = b;

== matlab function Tflex_PIDv1_ISSGP18a/Skewsine Setpoint Generator/Subsystem/MATLAB Function ==
  data: hm input; x output; tm input; t input; x_dot output; x_ddot output
function [x,x_dot,x_ddot] = skewSine(hm,tm,t)

if (t>=0) && (t<=tm)
    x      = hm/tm*t - hm/(2*pi)*sin(2*pi/tm*t);
    x_dot  = hm/tm - hm/tm*cos(2*pi/tm*t);
    x_ddot = 2*pi*hm/(tm^2)*sin(2*pi/tm*t);
else
    x      = hm;
    x_dot  = 0;
    x_ddot = 0;
end
